simulink model "chazhi"  (R2019b)
settings: Solver=VariableStepAuto  StartTime=0.0  StopTime=10.0  RelTol=1e-3
undefined symbols (not defined in the file or in its folder): CRB_dT, ENV_dtTaskBaseCtrlx4
settings Model: Creator=YJR  LastModifiedBy=YJR

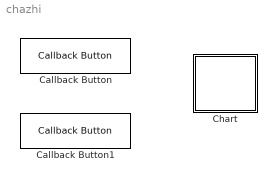
== system chazhi ==
  Callback Button : CallbackButton  ButtonText=POS1
      settings: ClickFcn=|
      | [DataList,~,~] = xlsread('abc','sheet2');
      | TimeList = DataList(:,1);
      | SpeedList = DataList(:,2);
      | assignin('base','CRB_dT',timeseries(SpeedList,TimeList));
  Callback Button1 : CallbackButton  ButtonText=POS2
      settings: ClickFcn=|
      | [DataList,~,~] = xlsread('abc','sheet2');
      | TimeList = DataList(:,1);
      | SpeedList = DataList(:,2);
      | assignin('base','ENV_dtTaskBaseCtrlx4',timeseries(SpeedList,TimeList));
  Chart : Stateflow chart  BlockKeywords=__PRM__SERIALIZED__DATA__:Stateflow Chart,Stateflow Diagram  TreatAsAtomicUnit=on

== stateflow chart chazhi/Chart ==
  state calc(in) [function]
    (default) -> (junction 2)
    (junction 2) -> (junction 13) : {delta_in=in-inK1;}
    (junction 13) -> (junction 15) [order 1] : [delta_in~=0]
    (junction 13) -> (junction 19) [order 2]
    (junction 15) -> (junction 17) : {
        | outK1=inK1;
        | delta_out=delta_in*CRB_dT/ENV_dtTaskBaseCtrlx4;
        | step=0;
        | }
    (junction 17) -> (junction 19)
    (junction 19) -> (junction 22)
    (junction 22) -> (junction 24) [order 1] : {step<(ENV_dtTaskBaseCtrlx4/CRB_dT-1)}
    (junction 22) -> (junction 46) [order 2] : {
        | out_=in
        | }
    (junction 24) -> (junction 26) : {
        | step = step + 1;
        | out_=outK1+delta_out;
        | }
    (junction 26) -> (junction 28) [order 1] : [delta_out<0]
    (junction 26) -> (junction 32) [order 2]
    (junction 28) -> (junction 30) : {
        | out_=max(out_,in);
        | }
    (junction 30) -> (junction 32)
    (junction 32) -> (junction 35)
    (junction 35) -> (junction 37) [order 1] : [delta_out>0]
    (junction 35) -> (junction 41) [order 2]
    (junction 37) -> (junction 39) : {
        | out_=min(out_,in);
        | }
    (junction 39) -> (junction 41)
    (junction 41) -> (junction 44)
    (junction 44) -> (junction 46)
    (junction 46) -> (junction 49) : {
        | inK1=in;
        | outK1=out_;
        | }
  data: in function_input double; step local; out_ local; delta_out local; delta_in local; ENV_dtTaskBaseCtrlx4 parameter single; CRB_dT parameter single; inK1 local; outK1 local
